simulink model "modelling1"  (R2021a)
settings: Solver=VariableStepAuto  StartTime=0.0  StopTime=1  FixedStep=1.0  RelTol=1e-9
libraries: simulink x6

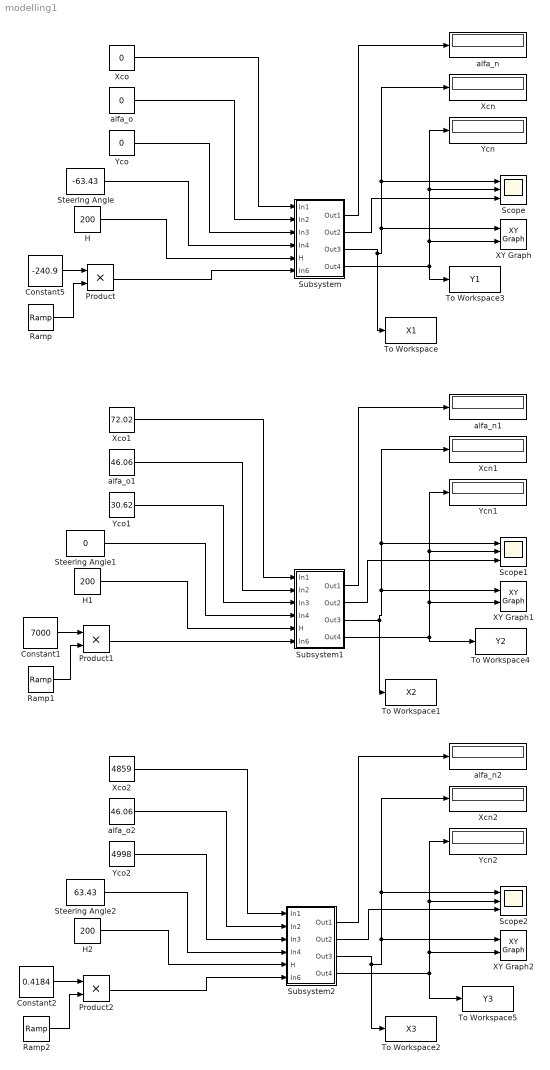
== system modelling1 ==
  Constant1 : Constant  Value=7000
  Constant2 : Constant  Value=0.4184
  Constant5 : Constant  Value=-240.9
  H : Constant  Value=200
  H1 : Constant  Value=200
  H2 : Constant  Value=200
  Product : Product
  Product1 : Product
  Product2 : Product
  Ramp : simulink/Sources/Ramp  slope=1  start=0  InitialOutput=0
  Ramp1 : simulink/Sources/Ramp  slope=1  start=0  InitialOutput=0
  Ramp2 : simulink/Sources/Ramp  slope=1  start=0  InitialOutput=0
  Scope : Scope  NumInputPorts=3
  Scope1 : Scope  NumInputPorts=3
  Scope2 : Scope  NumInputPorts=3
  Steering Angle : Constant  Value=-63.43
  Steering Angle1 : Constant  Value=0
  Steering Angle2 : Constant  Value=63.43
  Subsystem : Subsystem
  Subsystem1 : Subsystem
  Subsystem2 : Subsystem
  To Workspace : ToWorkspace  VariableName=X1  SampleTime=0.01
  To Workspace1 : ToWorkspace  VariableName=X2  SampleTime=0.01
  To Workspace2 : ToWorkspace  VariableName=X3  SampleTime=0.01
  To Workspace3 : ToWorkspace  VariableName=Y1  SampleTime=0.01
  To Workspace4 : ToWorkspace  VariableName=Y2  SampleTime=0.01
  To Workspace5 : ToWorkspace  VariableName=Y3  SampleTime=0.01
  XY Graph : simulink/Sinks/XY Graph  xmin=-500  xmax=500  ymin=-500  ymax=500  st=0.01
  XY Graph1 : simulink/Sinks/XY Graph  xmin=-1000  xmax=5200  ymin=-1000  ymax=5200  st=0.01
  XY Graph2 : simulink/Sinks/XY Graph  xmin=4000  xmax=5200  ymin=4000  ymax=5200  st=0.01
  Xcn : Display
  Xcn1 : Display
  Xcn2 : Display
  Xco : Constant  Value=0
  Xco1 : Constant  Value=72.02
  Xco2 : Constant  Value=4859
  Ycn : Display
  Ycn1 : Display
  Ycn2 : Display
  Yco : Constant  Value=0
  Yco1 : Constant  Value=30.62
  Yco2 : Constant  Value=4998
  alfa_n : Display
  alfa_n1 : Display
  alfa_n2 : Display
  alfa_o : Constant  Value=0
  alfa_o1 : Constant  Value=46.06
  alfa_o2 : Constant  Value=46.06
  wires:
  Subsystem/3(Out3) -> To Workspace/1, Xcn/1, Scope/1, XY Graph/1
  Subsystem/4(Out4) -> To Workspace3/1, XY Graph/2, Ycn/1, Scope/2
  Xco/1 -> Subsystem/1(In1)
  alfa_o/1 -> Subsystem/2(In2)
  Yco/1 -> Subsystem/3(In3)
  Steering Angle/1 -> Subsystem/4(In4)
  H/1 -> Subsystem/5(H)
  Product/1 -> Subsystem/6(In6)
  Subsystem/1(Out1) -> alfa_n/1
  Subsystem/2(Out2) -> Scope/3
  Subsystem1/2(Out2) -> Scope1/3
  H1/1 -> Subsystem1/5(H)
  Subsystem1/3(Out3) -> Xcn1/1, Scope1/1, XY Graph1/1, To Workspace1/1
  Subsystem1/1(Out1) -> alfa_n1/1
  Yco1/1 -> Subsystem1/3(In3)
  Subsystem1/4(Out4) -> XY Graph1/2, Ycn1/1, Scope1/2, To Workspace4/1
  alfa_o1/1 -> Subsystem1/2(In2)
  Steering Angle1/1 -> Subsystem1/4(In4)
  Xco1/1 -> Subsystem1/1(In1)
  Subsystem2/2(Out2) -> Scope2/3
  H2/1 -> Subsystem2/5(H)
  Subsystem2/1(Out1) -> alfa_n2/1
  Yco2/1 -> Subsystem2/3(In3)
  Subsystem2/4(Out4) -> To Workspace5/1, XY Graph2/2, Ycn2/1, Scope2/2
  alfa_o2/1 -> Subsystem2/2(In2)
  Steering Angle2/1 -> Subsystem2/4(In4)
  Xco2/1 -> Subsystem2/1(In1)
  Subsystem2/3(Out3) -> To Workspace2/1, Xcn2/1, Scope2/1, XY Graph2/1
  Ramp/1 -> Product/2
  Constant5/1 -> Product/1
  Ramp1/1 -> Product1/2
  Constant1/1 -> Product1/1
  Product1/1 -> Subsystem1/6(In6)
  Ramp2/1 -> Product2/2
  Constant2/1 -> Product2/1
  Product2/1 -> Subsystem2/6(In6)

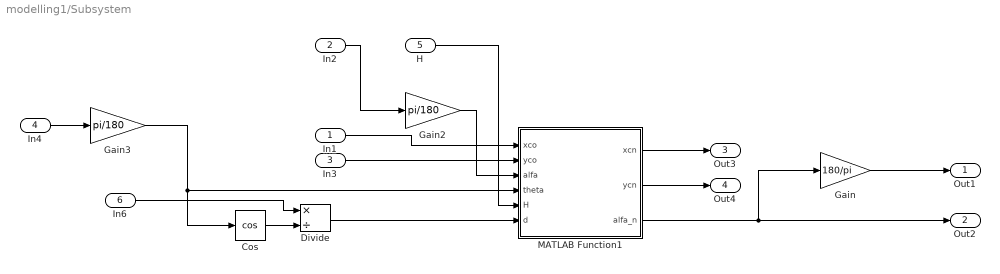
== system modelling1/Subsystem ==
  In1 : Inport
  In2 : Inport  Port=2
  In3 : Inport  Port=3
  In4 : Inport  Port=4
  H : Inport  Port=5
  In6 : Inport  Port=6
  Cos : Trigonometry  Operator=cos
  Divide : Product  Inputs=*/
  Gain : Gain  Gain=180/pi
  Gain2 : Gain  Gain=pi/180
  Gain3 : Gain  Gain=pi/180
  MATLAB Function1 : MATLAB Function  TreatAsAtomicUnit=on
  Out1 : Outport  VectorParamsAs1DForOutWhenUnconnected=off
  Out2 : Outport  Port=2  VectorParamsAs1DForOutWhenUnconnected=off
  Out3 : Outport  Port=3  VectorParamsAs1DForOutWhenUnconnected=off
  Out4 : Outport  Port=4  VectorParamsAs1DForOutWhenUnconnected=off
  wires:
  H/1 -> MATLAB Function1/5(H)
  In2/1 -> Gain2/1
  Gain3/1 -> MATLAB Function1/4(theta), Cos/1
  In4/1 -> Gain3/1
  Gain/1 -> Out1/1
  In3/1 -> MATLAB Function1/2(yco)
  Cos/1 -> Divide/2
  MATLAB Function1/2(ycn) -> Out4/1
  MATLAB Function1/3(alfa_n) -> Out2/1, Gain/1
  In6/1 -> Divide/1
  In1/1 -> MATLAB Function1/1(xco)
  MATLAB Function1/1(xcn) -> Out3/1
  Gain2/1 -> MATLAB Function1/3(alfa)
  Divide/1 -> MATLAB Function1/6(d)

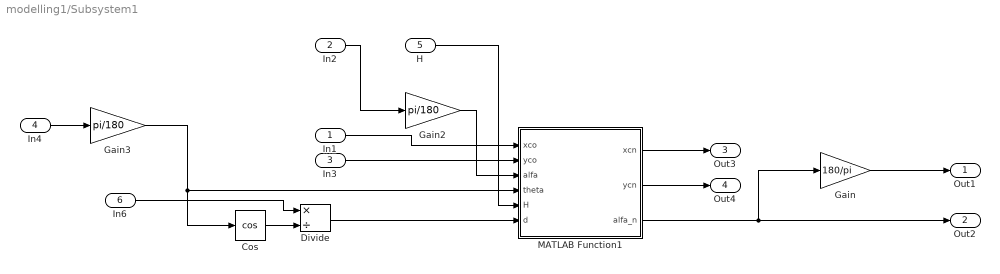
== system modelling1/Subsystem1 ==
  In1 : Inport
  In2 : Inport  Port=2
  In3 : Inport  Port=3
  In4 : Inport  Port=4
  H : Inport  Port=5
  In6 : Inport  Port=6
  Cos : Trigonometry  Operator=cos
  Divide : Product  Inputs=*/
  Gain : Gain  Gain=180/pi
  Gain2 : Gain  Gain=pi/180
  Gain3 : Gain  Gain=pi/180
  MATLAB Function1 : MATLAB Function  TreatAsAtomicUnit=on
  Out1 : Outport  VectorParamsAs1DForOutWhenUnconnected=off
  Out2 : Outport  Port=2  VectorParamsAs1DForOutWhenUnconnected=off
  Out3 : Outport  Port=3  VectorParamsAs1DForOutWhenUnconnected=off
  Out4 : Outport  Port=4  VectorParamsAs1DForOutWhenUnconnected=off
  wires:
  Gain2/1 -> MATLAB Function1/3(alfa)
  MATLAB Function1/1(xcn) -> Out3/1
  In1/1 -> MATLAB Function1/1(xco)
  In6/1 -> Divide/1
  MATLAB Function1/3(alfa_n) -> Out2/1, Gain/1
  Cos/1 -> Divide/2
  MATLAB Function1/2(ycn) -> Out4/1
  Divide/1 -> MATLAB Function1/6(d)
  In2/1 -> Gain2/1
  In4/1 -> Gain3/1
  Gain3/1 -> MATLAB Function1/4(theta), Cos/1
  In3/1 -> MATLAB Function1/2(yco)
  Gain/1 -> Out1/1
  H/1 -> MATLAB Function1/5(H)

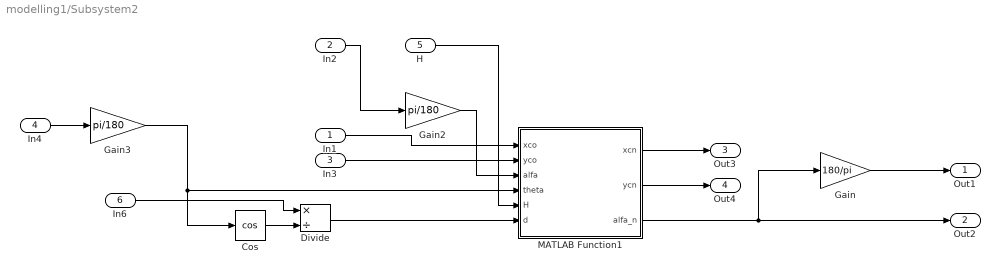
== system modelling1/Subsystem2 ==
  In1 : Inport
  In2 : Inport  Port=2
  In3 : Inport  Port=3
  In4 : Inport  Port=4
  H : Inport  Port=5
  In6 : Inport  Port=6
  Cos : Trigonometry  Operator=cos
  Divide : Product  Inputs=*/
  Gain : Gain  Gain=180/pi
  Gain2 : Gain  Gain=pi/180
  Gain3 : Gain  Gain=pi/180
  MATLAB Function1 : MATLAB Function  TreatAsAtomicUnit=on
  Out1 : Outport  VectorParamsAs1DForOutWhenUnconnected=off
  Out2 : Outport  Port=2  VectorParamsAs1DForOutWhenUnconnected=off
  Out3 : Outport  Port=3  VectorParamsAs1DForOutWhenUnconnected=off
  Out4 : Outport  Port=4  VectorParamsAs1DForOutWhenUnconnected=off
  wires:
  Gain2/1 -> MATLAB Function1/3(alfa)
  MATLAB Function1/1(xcn) -> Out3/1
  In1/1 -> MATLAB Function1/1(xco)
  In6/1 -> Divide/1
  MATLAB Function1/3(alfa_n) -> Out2/1, Gain/1
  Cos/1 -> Divide/2
  MATLAB Function1/2(ycn) -> Out4/1
  Divide/1 -> MATLAB Function1/6(d)
  In2/1 -> Gain2/1
  In4/1 -> Gain3/1
  Gain3/1 -> MATLAB Function1/4(theta), Cos/1
  In3/1 -> MATLAB Function1/2(yco)
  Gain/1 -> Out1/1
  H/1 -> MATLAB Function1/5(H)

== matlab function modelling1/Subsystem/MATLAB Function1 ==
function [xcn,ycn,alfa_n] = fcn(xco,yco,alfa,theta,H,d)
L=-H/cos((pi/2)-theta);
beta = d/L;
R = H *tan((pi/2)-theta);
gama = (((pi-beta)/2)-(alfa-pi/2));
alfa_n =(pi/2)+((alfa-pi/2)+beta) ;
xcn=xco+2*R*sin(beta/2)*cos(gama);
ycn=yco-2*R*sin(beta/2)*sin(gama);

== matlab function modelling1/Subsystem1/MATLAB Function1 ==
function [xcn,ycn,alfa_n] = fcn(xco,yco,alfa,theta,H,d)
L=-H/cos((pi/2)-theta);
beta = d/L;
R = H *tan((pi/2)-theta);
gama = (((pi-beta)/2)-(alfa-pi/2));
alfa_n =(pi/2)+((alfa-pi/2)+beta) ;
xcn=xco+2*R*sin(beta/2)*cos(gama);
ycn=yco-2*R*sin(beta/2)*sin(gama);

== matlab function modelling1/Subsystem2/MATLAB Function1 ==
function [xcn,ycn,alfa_n] = fcn(xco,yco,alfa,theta,H,d)
L=-H/cos((pi/2)-theta);
beta = d/L;
R = H *tan((pi/2)-theta);
gama = (((pi-beta)/2)-(alfa-pi/2));
alfa_n =(pi/2)+((alfa-pi/2)+beta) ;
xcn=xco+2*R*sin(beta/2)*cos(gama);
ycn=yco-2*R*sin(beta/2)*sin(gama);
